simulink model "MBKwithLQR"  (R2020a)
settings: Solver=ode4  StartTime=0.0  StopTime=10  FixedStep=0.01  RelTol=1e-3
InitFcn:
  | MBK
values from neighbouring files (symbols this model uses):
  b = 2    [riccati.m]
  k = 5    [riccati.m]
  m = 10    [riccati.m]
settings Model: PauseTimes=0  Creator=Ali  LastModifiedBy=Ali
settings DataIOCC: ReturnWorkspaceOutputs=off
settings DebuggingCC: ArithmeticOperatorsInVariantConditions=warning
settings SFSimCC: SimUseLocalCustomCode=off  CustomCodeUndefinedFunction=UseInterfaceOnly
settings RTWCC: RTWUseLocalCustomCode=off

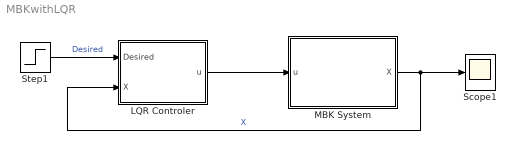
== system MBKwithLQR ==
  LQR Controler : Subsystem
  MBK System : Subsystem
  Scope1 : Scope
  Step1 : Step  After=6  SampleTime=0
  wires:
  MBK System/1(X) -> LQR Controler/2(X), Scope1/1  "X"
  Step1/1 -> LQR Controler/1(Desired)  "Desired"
  LQR Controler/1(u) -> MBK System/1(u)

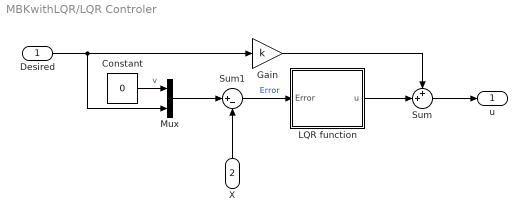
== system MBKwithLQR/LQR Controler ==
  Desired : Inport
  X : Inport  Port=2
  Constant : Constant  Value=0
  Gain : Gain  Gain=k
  LQR function : MATLAB Function  TreatAsAtomicUnit=on
  Mux : Mux  Inputs=2
  Sum : Sum  Inputs=++|
  Sum1 : Sum  Inputs=|+-
  u : Outport  VectorParamsAs1DForOutWhenUnconnected=off
  wires:
  X/1 -> Sum1/2
  Mux/1 -> Sum1/1
  LQR function/1(u) -> Sum/2
  Constant/1 -> Mux/1  "v"
  Sum/1 -> u/1
  Sum1/1 -> LQR function/1(Error)  "Error"
  Gain/1 -> Sum/1
  Desired/1 -> Gain/1, Mux/2

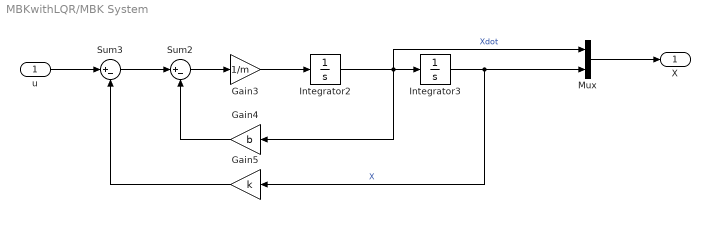
== system MBKwithLQR/MBK System ==
  u : Inport
  Gain3 : Gain  Gain=1/m
  Gain4 : Gain  Gain=b
  Gain5 : Gain  Gain=k
  Integrator2 : Integrator
  Integrator3 : Integrator  InitialCondition=3
  Mux : Mux  Inputs=2
  Sum2 : Sum  Inputs=|+-
  Sum3 : Sum  Inputs=|+-
  X : Outport  VectorParamsAs1DForOutWhenUnconnected=off
  wires:
  u/1 -> Sum3/1
  Gain4/1 -> Sum2/2
  Gain3/1 -> Integrator2/1
  Integrator3/1 -> Mux/2, Gain5/1  "X"
  Gain5/1 -> Sum3/2
  Sum2/1 -> Gain3/1
  Integrator2/1 -> Mux/1, Gain4/1, Integrator3/1  "Xdot"
  Sum3/1 -> Sum2/1
  Mux/1 -> X/1

== matlab function MBKwithLQR/LQR Controler/LQR function ==
  settings: updateMethod=DISCRETE
  data: u output; Error input
function u = LQR(Error)
m = 10;
b = 2;
k = 5;
A = [0    1;
   -k/m -b/m];
B = [0; 1/m];
Q = [2000 0;...
     0 10] ;
R = 1;
persistent Forloop;
persistent K_ans;
if isempty(Forloop)
    K_ans = zeros(2, 2);
    % algebraic_riccati = K * A + A' * K - K * B * R^-1 * B' * K + Q;
    % first equation - K12^2/m^2 - (2*K12*k)/m + Q11 = 0
    % Ans1 K12 = -m*(k + (k^2 + Q11)^(1/2))
    % Ans2 K12 = -m*(k - (k^2 + Q11)^(1/2))
    K12 = zeros(1, 2);
    K12(1) = -m*(k + (k^2 + Q(1, 1))^(1/2));
    K12(2) = -m*(k - (k^2 + Q(1, 1))^(1/2));
    for i = 1:length(K12)
        if ~isreal(K12(i))
            continue;
        end
        % Second equation 2*K12 + Q22 - K22^2/m^2 - (2*K22*b)/m = 0
        % Ans1 K12 = -m*(b + (b^2 + 2*K12 + Q22)^(1/2))
        % Ans2 K12 = -m*(b + (b^2 + 2*K12 + Q22)^(1/2))
        K22 = zeros(1, 2);
        K22(1) = -m*(b + (b^2 + 2*K12(i) + Q(2, 2))^(1/2));
        K22(2) = -m*(b - (b^2 + 2*K12(i) + Q(2, 2))^(1/2));
        for j = 1:length(K22)
            if ~isreal(K22(j))
                continue
            end
            % Last equation K11 - (K12*K22)/m^2 - (K12*b)/m - (K22*k)/m
            % Ans (K12*K22 + K12*b*m + K22*k*m)/m^2
            K11 = (K12(i)*K22(j) + K12(i)*b*m + K22(j)*k*m)/m^2;
            temp_K = zeros(2, 2);
            temp_K(1, 1) = K11;
            temp_K(1, 2) = K12(i);
            temp_K(2, 1) = K12(i);
            temp_K(2, 2) = K22(j);
            if all(eig(A - B * R^(-1)* B' * temp_K) < 0)
                Forloop = 1;
                K_ans = temp_K;
                break;
            end
        end
        if isempty(Forloop)
            break;
        end
    end
end
Temp = zeros(2, 1);
Temp(1) = Error(2, 1);
Temp(2) = Error(1, 1);
u_coefficient = -B * R^(-1)* B' *K_ans;
u = -u_coefficient*Temp;
